simulink model "main_sim"  (R2025b)
settings: Solver=VariableStepAuto  StartTime=0.0  StopTime=10.0  RelTol=1e-3
settings Model: Creator=flof  LastModifiedBy=2712f

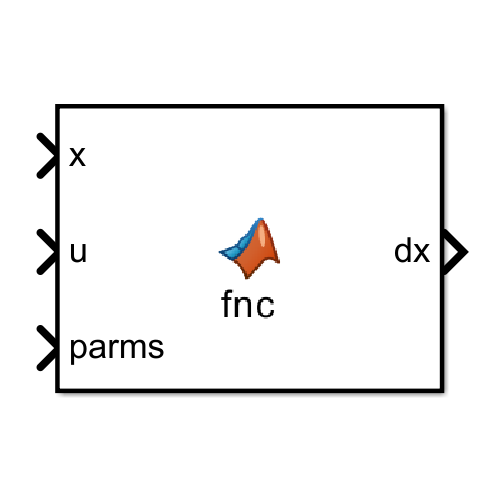
[thumbnail: Simulink's stored preview of the top-level diagram]
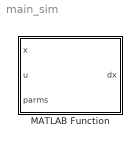
== system main_sim ==
  MATLAB Function : MATLAB Function  TreatAsAtomicUnit=on

== matlab function main_sim/MATLAB Function ==
  data: x input; dx output; u input; parms input
function dx = fnc(x,u,parms)

dx = f(x,parms) + g(x,u,parms);
